simulink model "dynamic_sim_II"  (R2016a)
settings: Solver=VariableStepAuto  StartTime=0.0  StopTime=1  RelTol=1e-3
values from neighbouring files (symbols this model uses):
  F = 1e-7    (= 1e-07)    [dynamic_sim_constants.m]
  J = 1e-9    (= 1e-09)    [dynamic_sim_constants.m]
  Ki_q = 0.00001    (= 1e-05)    [dynamic_sim_constants.m]
  Km = .00149    (= 0.00149)    [dynamic_sim_constants.m]
  Kp_q = 10    [dynamic_sim_constants.m]
  L = 0.00001462*3/2    (= 2.193e-05)    [dynamic_sim_constants.m]    (also in serial_bin_log.m = length(log))
  L_obs = L*err_gain    (= 2.4123e-05)    [dynamic_sim_constants.m]
  P = 2    [dynamic_sim_constants.m]    (also in foc_matlab_plot.m = mean(avg_st); serial_bin_log.m = mean(avg_st); slow_1hz_current_data_2_1A.mat = 0.00101490868431; slow_1hz_current_datas.mat = 0.00101490868431)
  psi = 0.00152788745    [dynamic_sim_constants.m]
  psi_obs = psi*err_gain    (= 0.001680676195)    [dynamic_sim_constants.m]
  R = .86*3/2    (= 1.29)    [dynamic_sim_constants.m]
  R_obs = R*err_gain    (= 1.419)    [dynamic_sim_constants.m]
settings Model: Creator=Ocanath  LastModifiedBy=Ocanath

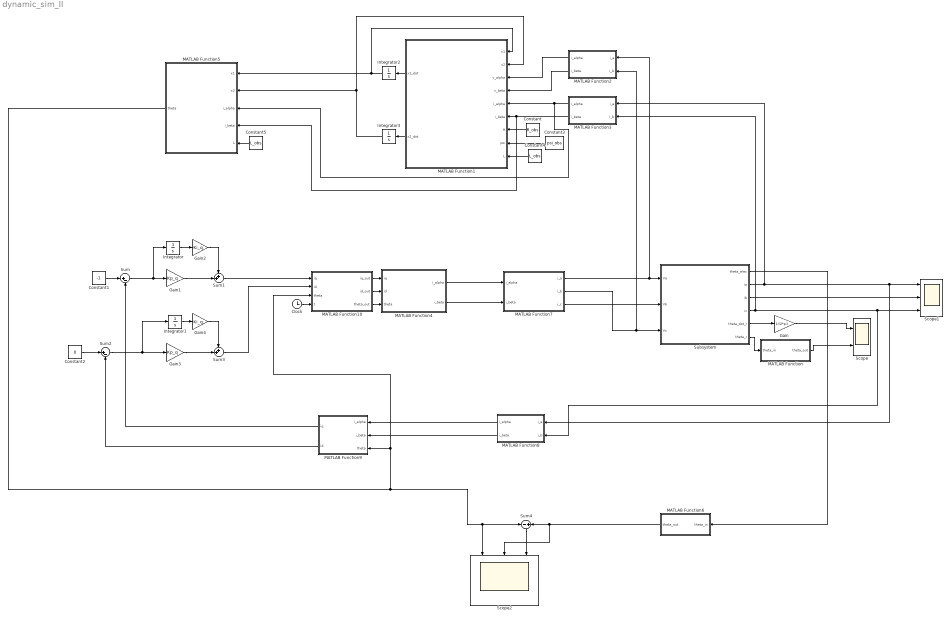
== system dynamic_sim_II ==
  Clock : Clock
      settings: Decimation=1000
  Constant : Constant  Value=R_obs
  Constant1 : Constant  Value=-1
  Constant2 : Constant  Value=0
  Constant3 : Constant  Value=psi_obs
  Constant4 : Constant  Value=L_obs
  Constant5 : Constant  Value=L_obs
  Gain : Gain  Gain=1/(2*pi)
  Gain1 : Gain  Gain=Kp_q
  Gain2 : Gain  Gain=Ki_q
  Gain3 : Gain  Gain=Kp_q
  Gain4 : Gain  Gain=Ki_q
  Integrator{,1..3} (4 alike) : Integrator
  MATLAB Function : MATLAB Function  TreatAsAtomicUnit=on
  MATLAB Function1 : MATLAB Function  TreatAsAtomicUnit=on
  MATLAB Function10 : MATLAB Function  TreatAsAtomicUnit=on
  MATLAB Function2 : MATLAB Function  TreatAsAtomicUnit=on
  MATLAB Function3 : MATLAB Function  TreatAsAtomicUnit=on
  MATLAB Function4 : MATLAB Function  TreatAsAtomicUnit=on
  MATLAB Function5 : MATLAB Function  TreatAsAtomicUnit=on
  MATLAB Function6 : MATLAB Function  TreatAsAtomicUnit=on
  MATLAB Function7 : MATLAB Function  TreatAsAtomicUnit=on
  MATLAB Function8 : MATLAB Function  TreatAsAtomicUnit=on
  MATLAB Function9 : MATLAB Function  TreatAsAtomicUnit=on
  Scope : Scope  NumInputPorts=2
  Scope1 : Scope  NumInputPorts=3
  Scope2 : Scope  NumInputPorts=3
  Subsystem : Subsystem
  Sum : Sum  Inputs=|+-
  Sum1 : Sum  Inputs=++|
  Sum2 : Sum  Inputs=|+-
  Sum3 : Sum  Inputs=++|
  Sum4 : Sum  Inputs=-+
  wires:
  MATLAB Function4/1(i_alpha) -> MATLAB Function7/1(i_alpha)
  MATLAB Function4/2(i_beta) -> MATLAB Function7/2(i_beta)
  MATLAB Function7/1(i_a) -> MATLAB Function2/1(i_a), Subsystem/1("Va ")
  Subsystem/4(ic) -> MATLAB Function3/2(i_b), Scope1/3, MATLAB Function8/2(i_b)
  Subsystem/5(theta_dot_r) -> Gain/1
  MATLAB Function8/2(i_beta) -> MATLAB Function9/2(i_beta)
  MATLAB Function8/1(i_alpha) -> MATLAB Function9/1(i_alpha)
  Subsystem/6(theta_r) -> MATLAB Function/1(theta_in)
  MATLAB Function/1(theta_out) -> Scope/2
  Gain/1 -> Scope/1
  MATLAB Function7/2(i_b) -> MATLAB Function2/2(i_b), Subsystem/3(Vc)
  MATLAB Function7/3(i_c) -> Subsystem/2(Vb)
  Subsystem/2(ia) -> MATLAB Function3/1(i_a), MATLAB Function8/1(i_a), Scope1/1
  Subsystem/3(ib) -> Scope1/2
  Constant1/1 -> Sum/1
  Sum/1 -> Integrator/1, Gain1/1
  Gain1/1 -> Sum1/2
  Integrator/1 -> Gain2/1
  Gain2/1 -> Sum1/1
  Constant2/1 -> Sum2/1
  Sum2/1 -> Integrator1/1, Gain3/1
  MATLAB Function9/2(id) -> Sum2/2
  Gain3/1 -> Sum3/2
  Integrator1/1 -> Gain4/1
  Gain4/1 -> Sum3/1
  MATLAB Function9/1(iq) -> Sum/2
  MATLAB Function1/1(x1_dot) -> Integrator2/1
  MATLAB Function1/2(x2_dot) -> Integrator3/1
  Integrator2/1 -> MATLAB Function5/1(x1), MATLAB Function1/1(x1)
  Integrator3/1 -> MATLAB Function5/2(x2), MATLAB Function1/2(x2)
  MATLAB Function2/1(i_alpha) -> MATLAB Function1/3(v_alpha)
  MATLAB Function2/2(i_beta) -> MATLAB Function1/4(v_beta)
  Constant/1 -> MATLAB Function1/7(R)
  Constant3/1 -> MATLAB Function1/8(psi)
  Constant4/1 -> MATLAB Function1/9(L)
  MATLAB Function3/1(i_alpha) -> MATLAB Function5/3(i_alpha), MATLAB Function1/5(i_alpha)
  MATLAB Function3/2(i_beta) -> MATLAB Function5/4(i_beta), MATLAB Function1/6(i_beta)
  Constant5/1 -> MATLAB Function5/5(L)
  Sum4/1 -> Scope2/3
  Subsystem/1(" theta_elec ") -> MATLAB Function6/1(theta_in)
  Sum1/1 -> MATLAB Function10/1(iq)
  Sum3/1 -> MATLAB Function10/2(id)
  MATLAB Function6/1(theta_out) -> Scope2/2, Sum4/2
  MATLAB Function5/1(theta) -> Scope2/1, Sum4/1, MATLAB Function10/3(theta), MATLAB Function9/3(theta)
  MATLAB Function10/3(theta_out) -> MATLAB Function4/3(theta)
  MATLAB Function10/2(id_out) -> MATLAB Function4/2(id)
  MATLAB Function10/1(iq_out) -> MATLAB Function4/1(iq)
  Clock/1 -> MATLAB Function10/4(t)

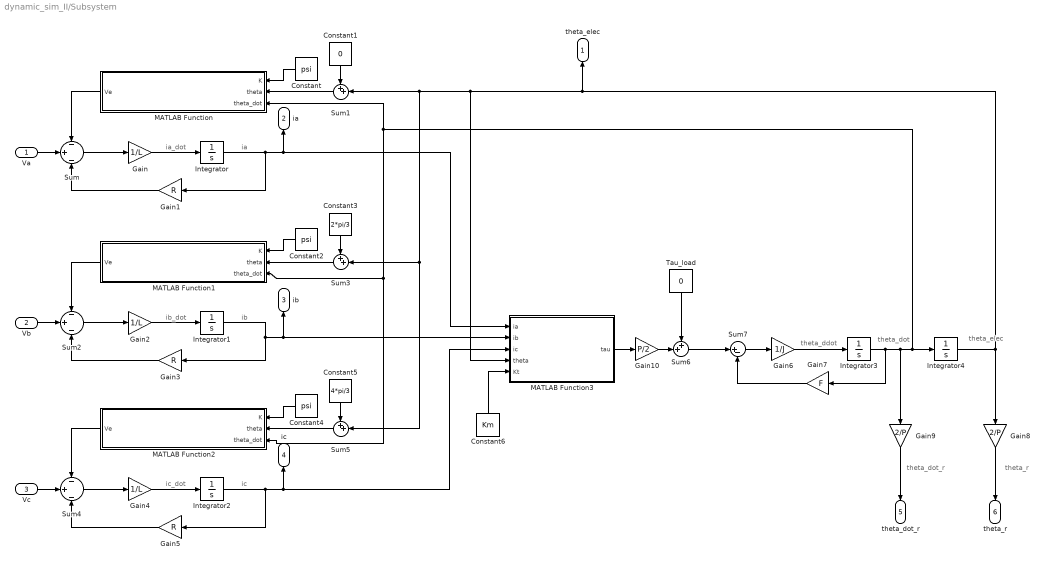
== system dynamic_sim_II/Subsystem ==
  note: theta_dot_r
  note: theta_r
  note: theta_elec
  note: theta_dot
  note: theta_ddot
  note: ia
  note: ia_dot
  note: ib
  note: ib_dot
  note: ic
  note: ic_dot
  "Va " : Inport
  Vb : Inport  Port=2
  Vc : Inport  Port=3
  Constant : Constant  Value=psi
  Constant1 : Constant  Value=0
  Constant2 : Constant  Value=psi
  Constant3 : Constant  Value=2*pi/3
  Constant4 : Constant  Value=psi
  Constant5 : Constant  Value=4*pi/3
  Constant6 : Constant  Value=Km
  Gain : Gain  Gain=1/L
  Gain1 : Gain  Gain=R
  Gain10 : Gain  Gain=P/2
  Gain2 : Gain  Gain=1/L
  Gain3 : Gain  Gain=R
  Gain4 : Gain  Gain=1/L
  Gain5 : Gain  Gain=R
  Gain6 : Gain  Gain=1/J
  Gain7 : Gain  Gain=F
  Gain8 : Gain  Gain=2/P
  Gain9 : Gain  Gain=2/P
  Integrator{,1..4} (5 alike) : Integrator
  MATLAB Function : MATLAB Function  TreatAsAtomicUnit=on
  MATLAB Function1 : MATLAB Function  TreatAsAtomicUnit=on
  MATLAB Function2 : MATLAB Function  TreatAsAtomicUnit=on
  MATLAB Function3 : MATLAB Function  TreatAsAtomicUnit=on
  Sum : Sum  Inputs=-|+|-
  Sum{1,3,5..6} (4 alike) : Sum  Inputs=++|
  Sum2 : Sum  Inputs=-|+|-
  Sum4 : Sum  Inputs=-|+|-
  Sum7 : Sum  Inputs=|+-
  Tau_load : Constant  Value=0
  " theta_elec " : Outport
  ia : Outport  Port=2
  ib : Outport  Port=3
  ic : Outport  Port=4
  theta_dot_r : Outport  Port=5
  theta_r : Outport  Port=6
  wires:
  Gain4/1 -> Integrator2/1
  Sum6/1 -> Sum7/1
  Sum5/1 -> MATLAB Function2/2(theta)
  Gain5/1 -> Sum4/3
  Integrator4/1 -> " theta_elec "/1, MATLAB Function3/4(theta), Sum5/2, Sum3/2, Sum1/2, Gain8/1
  Sum4/1 -> Gain4/1
  Integrator/1 -> Gain1/1, ia/1, MATLAB Function3/1(ia)
  Constant6/1 -> MATLAB Function3/5(Kt)
  Integrator2/1 -> Gain5/1, ic/1, MATLAB Function3/3(ic)
  Gain/1 -> Integrator/1
  MATLAB Function1/1(Ve) -> Sum2/1
  Sum2/1 -> Gain2/1
  Gain2/1 -> Integrator1/1
  MATLAB Function2/1(Ve) -> Sum4/1
  Gain3/1 -> Sum2/3
  Sum1/1 -> MATLAB Function/2(theta)
  Integrator1/1 -> Gain3/1, ib/1, MATLAB Function3/2(ib)
  Constant/1 -> MATLAB Function/1(K)
  Constant2/1 -> MATLAB Function1/1(K)
  Constant3/1 -> Sum3/1
  Gain1/1 -> Sum/3
  Sum/1 -> Gain/1
  Constant4/1 -> MATLAB Function2/1(K)
  Integrator3/1 -> MATLAB Function2/3(theta_dot), MATLAB Function1/3(theta_dot), MATLAB Function/3(theta_dot), Integrator4/1, Gain9/1, Gain7/1
  Constant1/1 -> Sum1/1
  Sum3/1 -> MATLAB Function1/2(theta)
  Constant5/1 -> Sum5/1
  MATLAB Function3/1(tau) -> Gain10/1
  MATLAB Function/1(Ve) -> Sum/1
  Tau_load/1 -> Sum6/1
  Gain8/1 -> theta_r/1
  Sum7/1 -> Gain6/1
  Gain6/1 -> Integrator3/1
  Gain9/1 -> theta_dot_r/1
  Vc/1 -> Sum4/2
  Vb/1 -> Sum2/2
  "Va "/1 -> Sum/2
  Gain7/1 -> Sum7/2
  Gain10/1 -> Sum6/2

== matlab function dynamic_sim_II/Subsystem/MATLAB Function1 ==
  data: K input; Ve output; theta input; theta_dot input
function Ve = emf(K,theta,theta_dot)
%#codegen
Ve = K*sin(theta)*theta_dot;
end

== matlab function dynamic_sim_II/Subsystem/MATLAB Function ==
  data: K input; Ve output; theta input; theta_dot input
function Ve = emf(K,theta,theta_dot)
%#codegen
Ve = K*sin(theta)*theta_dot;
end

== matlab function dynamic_sim_II/Subsystem/MATLAB Function2 ==
  data: K input; Ve output; theta input; theta_dot input
function Ve = emf(K,theta,theta_dot)
%#codegen
Ve = K*sin(theta)*theta_dot;
end

== matlab function dynamic_sim_II/Subsystem/MATLAB Function3 ==
  data: ia input; tau output; ib input; ic input; theta input; Kt input
function tau = tau_elec(ia,ib,ic,theta,Kt)

tau = Kt*(ia*sin(theta) + ib*sin(theta+2*pi/3) + ic*sin(theta+4*pi/3));

end

== matlab function dynamic_sim_II/MATLAB Function4 ==
  data: iq input; i_alpha output; id input; theta input; i_beta output
function [i_alpha,i_beta] = inverse_park(iq, id, theta)
    sin_theta = sin(theta);
    cos_theta = cos(theta);
    i_alpha = id*cos_theta - iq*sin_theta;
	i_beta = id*sin_theta + iq*cos_theta;
end

== matlab function dynamic_sim_II/MATLAB Function ==
  data: theta_in input; theta_out output
function theta_out = encoder(theta_in)
theta_out = atan2(sin(theta_in),cos(theta_in));
end

== matlab function dynamic_sim_II/MATLAB Function1 ==
  data: x1 input; x2 input; v_alpha input; v_beta input; i_alpha input; x1_dot output; i_beta input; x2_dot output; R input; psi input; L input
function [x1_dot, x2_dot] = observer_state(x1, x2, v_alpha, v_beta, i_alpha, i_beta, R, psi, L)
n1 = x1 - L*i_alpha;
n2 = x2 - L*i_beta;

y1 = -R*i_alpha + v_alpha;
y2 = -R*i_beta + v_beta;

err = (psi*psi - (n1*n1 + n2*n2));

gamma = 100000000;

x1_dot = y1 + (gamma/2)*n1*err;
x2_dot = y2 + (gamma/2)*n2*err;

end

== matlab function dynamic_sim_II/MATLAB Function7 ==
  data: i_alpha input; i_a output; i_beta input; i_b output; i_c output
function [i_a,i_b,i_c] = inverse_clarke(i_alpha,i_beta)
    sqrt_3_by_2 = sqrt(3)*.5;
	i_a = i_alpha;
	i_b = -.5*i_alpha + sqrt_3_by_2*i_beta;
	i_c = -.5*i_alpha - sqrt_3_by_2*i_beta;
end

== matlab function dynamic_sim_II/MATLAB Function8 ==
  data: i_a input; i_alpha output; i_b input; i_beta output
function [i_alpha, i_beta] = clarke(i_a, i_b)
    i_alpha = i_a;
	i_beta = (1/sqrt(3))*i_a + (2/sqrt(3))*i_b;
end

== matlab function dynamic_sim_II/MATLAB Function9 ==
  data: i_alpha input; iq output; i_beta input; theta input; id output
function [iq,id] = park(i_alpha, i_beta, theta)
    cos_theta = cos(theta);
    sin_theta = sin(theta);
	id = i_alpha*cos_theta+i_beta*sin_theta;
	iq = -i_alpha*sin_theta+i_beta*cos_theta;
end

== matlab function dynamic_sim_II/MATLAB Function2 ==
  data: i_a input; i_alpha output; i_b input; i_beta output
function [i_alpha, i_beta] = clarke(i_a, i_b)
    i_alpha = i_a;
	i_beta = (1/sqrt(3))*i_a + (2/sqrt(3))*i_b;
end

== matlab function dynamic_sim_II/MATLAB Function3 ==
  data: i_a input; i_alpha output; i_b input; i_beta output
function [i_alpha, i_beta] = clarke(i_a, i_b)
    i_alpha = i_a;
	i_beta = (1/sqrt(3))*i_a + (2/sqrt(3))*i_b;
end

== matlab function dynamic_sim_II/MATLAB Function5 ==
  data: x1 input; theta output; x2 input; i_alpha input; i_beta input; L input
function theta = pos_estimator(x1,x2, i_alpha, i_beta, L)
theta = atan2( -(x2-L*i_beta), -(x1-L*i_alpha));
end

== matlab function dynamic_sim_II/MATLAB Function6 ==
  data: theta_in input; theta_out output
function theta_out = encoder(theta_in)
theta_out = atan2(sin(theta_in),cos(theta_in));
end

== matlab function dynamic_sim_II/MATLAB Function10 ==
  data: iq input; iq_out output; id input; theta input; t input; id_out output; theta_out output
function [iq_out,id_out,theta_out] = t_sw(iq,id,theta,t)
%#codegen
    iq_out = iq;
    id_out = id;
    theta_out = theta;
    if(t < .005)
        iq_out = -1;
        id_out = 0;
        theta_out = 2*pi*50*t;
    end
end
